simulink model "SimulinkCompensadores"  (R2020b)
settings: Solver=VariableStepAuto  StartTime=0.0  StopTime=95  RelTol=1e-3
undefined symbols (not defined in the file or in its folder): KI, KP
libraries: cstblocks x3
settings Model: Creator=sramirez  LastModifiedBy=sramirez

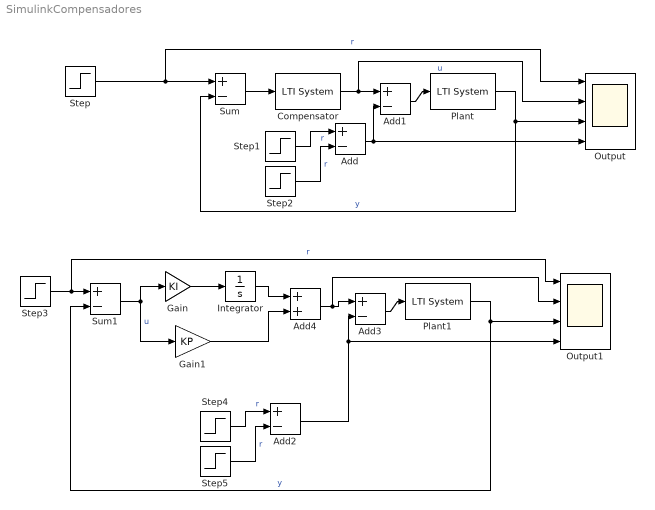
== system SimulinkCompensadores ==
  Add{,1..3} (4 alike) : Sum  Inputs=+-
  Add4 : Sum
  Compensator : cstblocks/LTI System  sys=C  IC=[]
  Gain : Gain  Gain=KI
  Gain1 : Gain  Gain=KP
  Integrator : Integrator
  Output : Scope  NumInputPorts=4
  Output1 : Scope  NumInputPorts=4
  Plant : cstblocks/LTI System  sys=G  IC=[]
  Plant1 : cstblocks/LTI System  sys=G  IC=[]
  Step : Step  Time=0  SampleTime=0
  Step1 : Step  Time=30  After=0.1  SampleTime=0
  Step2 : Step  Time=50  After=0.1  SampleTime=0
  Step3 : Step  Time=0.1  After=4  SampleTime=0
  Step4 : Step  Time=0.7  SampleTime=0
  Step5 : Step  Time=1.2  SampleTime=0
  Sum : Sum  Inputs=+-
  Sum1 : Sum  Inputs=+-
  wires:
  Step/1 -> Output/1, Sum/1  "r"
  Step2/1 -> Add/2  "r"
  Add3/1 -> Plant1/1
  Sum1/1 -> Gain1/1, Gain/1  "u"
  Plant/1 -> Output/3, Sum/2  "y"
  Add1/1 -> Plant/1
  Compensator/1 -> Output/2, Add1/1  "u"
  Step4/1 -> Add2/1  "r"
  Add4/1 -> Output1/2, Add3/1
  Integrator/1 -> Add4/1
  Gain1/1 -> Add4/2
  Step1/1 -> Add/1  "r"
  Add/1 -> Output/4, Add1/2
  Step5/1 -> Add2/2  "r"
  Gain/1 -> Integrator/1
  Sum/1 -> Compensator/1
  Plant1/1 -> Sum1/2, Output1/3  "y"
  Add2/1 -> Add3/2, Output1/4
  Step3/1 -> Sum1/1, Output1/1  "r"
